simulink model "Simple_3_Model_C"  (R2022b)
settings: Solver=FixedStepAuto  StartTime=0.0  StopTime=1000  FixedStep=.05  RelTol=1e-3
libraries: realtime_pacer_lib x1, ros2lib x1
settings Model: Creator=hollis  LastModifiedBy=hunter
settings OptimizationCC: DefaultParameterBehavior=Inlined  EnhancedBackFolding=on  PassReuseOutputArgsAs=Individual arguments  ZeroExternalMemoryAtStartup=off  ZeroInternalMemoryAtStartup=off  OptimizeBlockOrder=speed  DifferentSizesBufferReuse=on  OptimizationCustomize=off  EfficientTunableParamExpr=on
settings DebuggingCC: ParameterTunabilityLossMsg=error
settings HardwareCC: TargetBitPerLong=64  TargetBitPerPointer=64  TargetBitPerSizeT=64  TargetBitPerPtrDiffT=64  TargetLongLongMode=on  TargetIntDivRoundTo=Zero  TargetEndianess=LittleEndian  TargetWordSize=64  TargetHWDeviceType=MATLAB Host  ProdEqTarget=off
settings ModelReferenceCC: EnableRefExpFcnMdlSchedulingChecks=on
settings SFSimCC: MATLABDynamicMemAlloc=off  SimTargetLang=C++
settings RTWCC: Description=Embedded Coder (host-based shared library target)  SystemTargetFile=ert_shrlib.tlc  TemplateMakefile=ert_default_tmf  Toolchain=GNU gcc/g++ | CMake/gmake (64-bit Linux)  BuildConfiguration=Release
settings CodeAppCC: ForceParamTrailComments=on  IgnoreCustomStorageClasses=off  OperatorAnnotations=on  SimulinkDataObjDesc=on  SFDataObjDesc=on  InsertBlockDesc=on
settings STFCustomTargetCC: TargetLangStandard=C99 (ISO)  MultiwordLength=256  GenerateSampleERTMain=on  ParMdlRefBuildCompliant=on  CompOptLevelCompliant=on  CombineOutputUpdateFcns=on  ERTCustomFileBanners=on  SupportNonInlinedSFcns=off  RemoveResetFunc=on  MATLABClassNameForMDSCustomization=Simulink.SoftwareTarget.ERTCustomization  ModelStepFunctionPrototypeControlCompliant=on  UseToolchainInfoCompliant=on  SystemTargetFile=ert_shrlib.tlc
settings ERTTargetCC: TargetLangStandard=C99 (ISO)  GenerateSampleERTMain=on  ConcurrentExecutionCompliant=off  SupportContinuousTime=on  CPPClassGenCompliant=off  InlinedParameterPlacement=NonHierarchical  ERTCustomFileTemplate=example_file_process.tlc

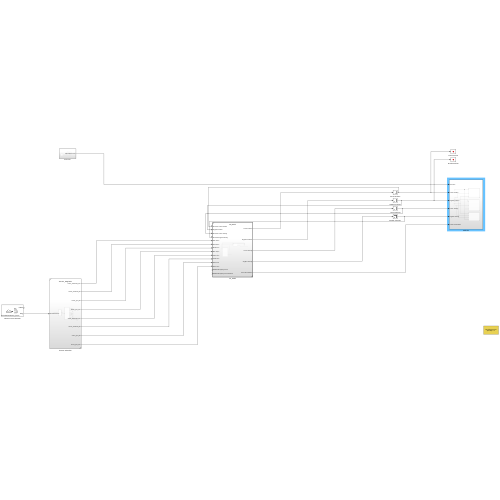
[thumbnail: Simulink's stored preview of the top-level diagram]
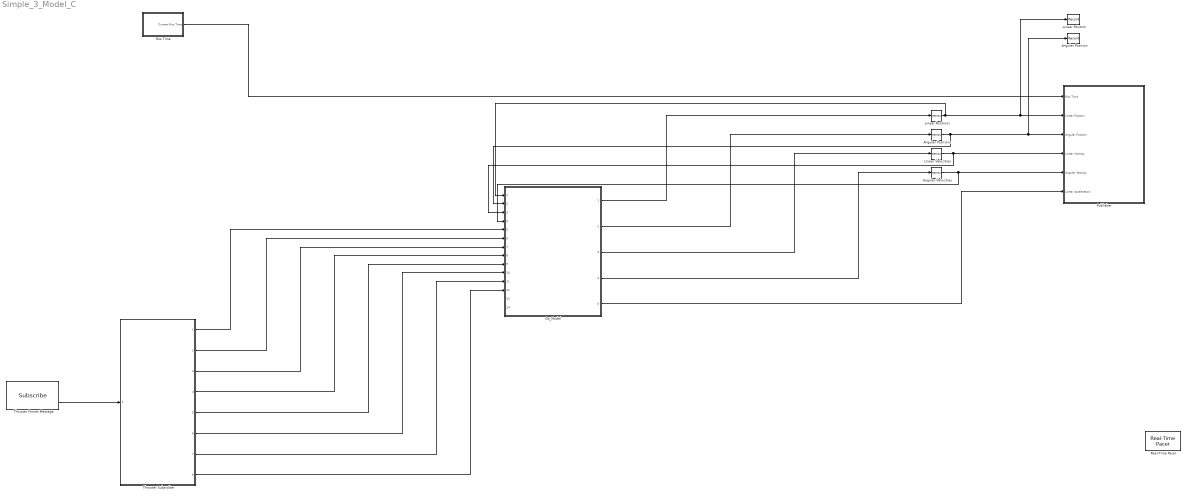
== system Simple_3_Model_C ==
  Angular Position : Record  FileSettingsInternal="{\"entries\":[{\"content\":{\"excelSettings\":{\"content\":{},\"type\":\"Streamout.ExcelSettings\"}},\"type\":\"Streamout.FileSettingStorage\",\"uuid\":\"5e6faace-5e05-446f-81ba-11f57939d993\"}],\"packageUris\":[\"http://schema.mathworks.com/mf0/streamout_blocks/R2020a\"],\"version\":\"1.0\"}"  SignalsInternal="{\"entries\":[{\"content\":{\"signals\":[{\"content\":{\"blockPath\":[\"Simple_3_Model_C/Angular Position\"],\"channel\":[],\"dimensions\":[1,3],\"domain\":\"Simple_3_Model_C/Angular Position\",\"hasChildren\":true,\"lineColor\":\"#b746ff\",\"plots\":[],\"port\":1,\"sid\":[],\"signalID\":309,\"signalName\":\"Angular Positions\"},\"type\":\"RecordBlkView.Signal\",\"uuid\":\"71cf2b88-9897-4e33-ab06-cf655d5c069d\"},{\"content\":{\"blockPath\":[\"Simple_3_Model_C/Angular Position\"],\"channel\":[1,1],\"dimensions\":[1,3],\"domain\":\"Simple_3_Model_C/Angular Position\",\"lineColor\":\"#d95319\",\"parentID\":309,\"plots\":[1],\"port\":1,\"sid\":[],\"signalID\":310,\"signalName\":\"Angular Positions\"},\"type\":\"RecordBlkView.Signal\",\"uuid\":\"81539e1a-8bab-4067-a60e-8d6090882496\"},{\"content\":{\"blockPath\":[\"Simple_3_Model_C/Angular Position\"],\"channel\":[1,2],\"dimensions\":[1,3],\"domain\":\"Simple_3_Model_C/Angular Position\",\"lineColor\":\"#d95319\",\"parentID\":309,\"plots\":[1],\"port\":1,\"sid\":[],\"signalID\":311,\"signalName\":\"Angular Positions\"},\"type\":\"RecordBlkView.Signal\",\"uuid\":\"9fdc422a-a8c8-4533-b613-6f9428fc65bd\"},{\"content\":{\"blockPath\":[\"Simple_3_Model_C/Angular Position\"],\"channel\":[1,3],\"dimensions\":[1,3],\"domain\":\"Simple_3_Model_C/Angular Position\",\"lineColor\":\"#edb120\",\"parentID\":309,\"plots\":[1],\"port\":1,\"sid\":[],\"signalID\":312,\"signalName\":\"Angular Positions\"},\"type\":\"RecordBlkView.Signal\",\"uuid\":\"9d0a805d-4d88-48d1-b17c-de63ad448efc\"}]},\"type\":\"RecordBlkView.InputSignals\",\"uuid\":\"3c6d1903-151d-4815-9e37-912ee027f4eb\"}],\"packageUris\":[\"http://schema.mathworks.com/mf0/streamout_blocks/R2020a\"],\"version\":\"1.0\"}"  VisualizationBindings="{\"sparklinesplugin\":{\"info\":[{\"bindingParametersList\":[],\"subplotID\":1}]}}"
  Angular Positions : Memory
  Angular Velocities : Memory
  Do_Model : Subsystem  TreatAsAtomicUnit=on  ReferencedSubsystem=Do_Model
  Linear Position : Record  FileSettingsInternal="{\"entries\":[{\"content\":{\"excelSettings\":{\"content\":{},\"type\":\"Streamout.ExcelSettings\"}},\"type\":\"Streamout.FileSettingStorage\",\"uuid\":\"9b40ccc1-229c-42d4-ab33-3394c1702d6d\"}],\"packageUris\":[\"http://schema.mathworks.com/mf0/streamout_blocks/R2020a\"],\"version\":\"1.0\"}"  SignalsInternal="{\"entries\":[{\"content\":{\"signals\":[{\"content\":{\"blockPath\":[\"Simple_3_Model_C/Linear Position\"],\"channel\":[],\"dimensions\":[1,3],\"domain\":\"Simple_3_Model_C/Linear Position\",\"hasChildren\":true,\"lineColor\":\"#ff13a6\",\"plots\":[],\"port\":1,\"sid\":[],\"signalID\":298,\"signalName\":\"Linear Positions\"},\"type\":\"RecordBlkView.Signal\",\"uuid\":\"238dd450-82a9-4540-9534-5454e0a4f67d\"},{\"content\":{\"blockPath\":[\"Simple_3_Model_C/Linear Position\"],\"channel\":[1,1],\"dimensions\":[1,3],\"domain\":\"Simple_3_Model_C/Linear Position\",\"lineColor\":\"#7e2f8e\",\"parentID\":298,\"plots\":[1],\"port\":1,\"sid\":[],\"signalID\":299,\"signalName\":\"Linear Positions\"},\"type\":\"RecordBlkView.Signal\",\"uuid\":\"0ffe9376-259a-4d51-9739-a81e551435e9\"},{\"content\":{\"blockPath\":[\"Simple_3_Model_C/Linear Position\"],\"channel\":[1,2],\"dimensions\":[1,3],\"domain\":\"Simple_3_Model_C/Linear Position\",\"lineColor\":\"#7e2f8e\",\"parentID\":298,\"plots\":[1],\"port\":1,\"sid\":[],\"signalID\":300,\"signalName\":\"Linear Positions\"},\"type\":\"RecordBlkView.Signal\",\"uuid\":\"2c7a0081-bf1d-46bd-8c42-e76470ee59e9\"},{\"content\":{\"blockPath\":[\"Simple_3_Model_C/Linear Position\"],\"channel\":[1,3],\"dimensions\":[1,3],\"domain\":\"Simple_3_Model_C/Linear Position\",\"lineColor\":\"#77ac30\",\"parentID\":298,\"plots\":[1],\"port\":1,\"sid\":[],\"signalID\":301,\"signalName\":\"Linear Positions\"},\"type\":\"RecordBlkView.Signal\",\"uuid\":\"79746674-a78a-4ff5-a75c-86a9df6f6110\"}]},\"type\":\"RecordBlkView.InputSignals\",\"uuid\":\"0a6c3fce-bcd9-43ed-9bd3-a9e2f38033f2\"}],\"packageUris\":[\"http://schema.mathworks.com/mf0/streamout_blocks/R2020a\"],\"version\":\"1.0\"}"  VisualizationBindings="{\"sparklinesplugin\":{\"info\":[{\"bindingParametersList\":[],\"subplotID\":1}]}}"
  Linear Positions : Memory  InitialCondition=[0.0,0.0,-1.0]
  Linear Velocities : Memory
  Publisher : Subsystem
  Real-Time Pacer : realtime_pacer_lib/Real-Time Pacer  simTimePerRealTime=1
  Ros Time : Subsystem
  Thruster Forces Message : ros2lib/Subscribe  topicSource=Specify your own  topic=/tempest/simulation/thruster_forces  messageType=std_msgs/Float32MultiArray  sampleTime=-1  QOSHistory=Keep last  QOSDepth=1  QOSReliability=Reliable  QOSDurability=Volatile
      settings: LibrarySourceBlock=roslib/ROS 2/Subscribe
  Thruster Subsrciber : Subsystem  ReferencedSubsystem=Thruster_Magnitude
  wires:
  Angular Velocities/1 -> Do_Model/4, Publisher/5(Angular Velocity)
  Linear Positions/1 -> Do_Model/1, Linear Position/1, Publisher/2(Linear Position)
  Linear Velocities/1 -> Do_Model/3, Publisher/4(Linear Velocity)
  Angular Positions/1 -> Do_Model/2, Angular Position/1, Publisher/3(Angular Position)
  Ros Time/1(Current Ros Time) -> Publisher/1(Ros Time)
  Thruster Forces Message/2 -> Thruster Subsrciber/1
  Thruster Subsrciber/1 -> Do_Model/5
  Thruster Subsrciber/2 -> Do_Model/6
  Thruster Subsrciber/3 -> Do_Model/7
  Thruster Subsrciber/4 -> Do_Model/8
  Thruster Subsrciber/5 -> Do_Model/9
  Thruster Subsrciber/6 -> Do_Model/10
  Thruster Subsrciber/7 -> Do_Model/11
  Thruster Subsrciber/8 -> Do_Model/12
  Do_Model/1 -> Linear Positions/1
  Do_Model/2 -> Angular Positions/1
  Do_Model/3 -> Linear Velocities/1
  Do_Model/4 -> Angular Velocities/1
  Do_Model/5 -> Publisher/6(Linear Acceleration)

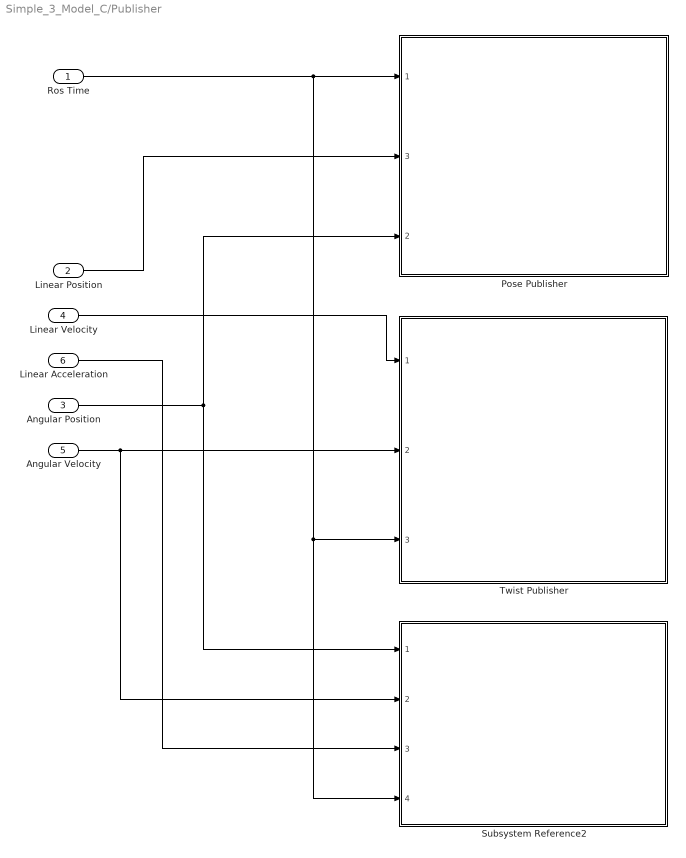
== system Simple_3_Model_C/Publisher ==
  Ros Time : Inport
  Linear Position : Inport  Port=2
  Angular Position : Inport  Port=3
  Linear Velocity : Inport  Port=4
  Angular Velocity : Inport  Port=5
  Linear Acceleration : Inport  Port=6
  Pose Publisher : Subsystem  ReferencedSubsystem=Pose_Publisher
      settings: PortSchema="{\"entries\":[{\"content\":{\"sides\":[{\"content\":{\"connectorIds\":[\"In1\",\"In3\",\"In2\"]},\"type\":\"ConnectorPlacement.EquallySpacedRectSide\",\"uuid\":\"18965d15-4955-4736-88eb-98a03933ea40\"},{\"content\":{\"connectorIds\":[],\"side\":\"RIGHT\"},\"type\":\"ConnectorPlacement.EquallySpacedRectSide\",\"uuid\":\"0239975c-7916-4f79-8798-13edb7247875\"},{\"content\":{\"connectorIds\":[],\"side\":\"TOP\"},\"type\":\"ConnectorPlacement.EquallySpacedRectSide\",\"uuid\":\"c7399201-5872-4101-b484-2a6e35d6576e\"}]},\"type\":\"ConnectorPlacement.EquallySpacedConnector\",\"uuid\":\"5ae7f81e-60af-4dbc-8d3d-d59049f94250\"}],\"packageUris\":[\"http://schema.mathworks.com/mf0/Connector/R2020b\"],\"version\":\"1.0\"}"
  Subsystem Reference2 : Subsystem  ReferencedSubsystem=Imu_Publisher
  Twist Publisher : Subsystem  ReferencedSubsystem=Twist_Publisher
  wires:
  Linear Position/1 -> Pose Publisher/3
  Linear Velocity/1 -> Twist Publisher/1
  Angular Position/1 -> Pose Publisher/2, Subsystem Reference2/1
  Angular Velocity/1 -> Subsystem Reference2/2, Twist Publisher/2
  Linear Acceleration/1 -> Subsystem Reference2/3
  Ros Time/1 -> Twist Publisher/3, Subsystem Reference2/4, Pose Publisher/1

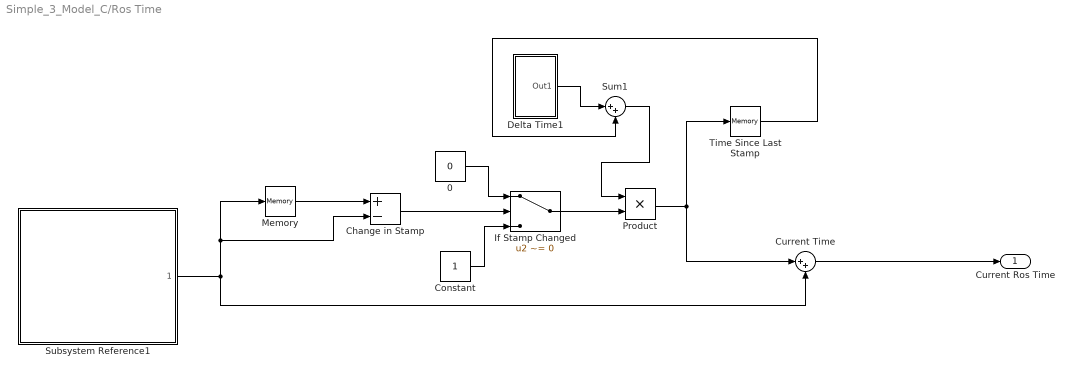
== system Simple_3_Model_C/Ros Time ==
  0 : Constant  Value=0
  Change in Stamp : Sum  Inputs=+-
  Constant : Constant
  Current Time : Sum  Inputs=|++
  Delta Time1 : Subsystem
  If Stamp Changed : Switch  Criteria=u2 ~= 0  SaturateOnIntegerOverflow=off  InputSameDT=off
  Memory : Memory
  Product : Product
  Subsystem Reference1 : Subsystem  ReferencedSubsystem=TimeSubscriber
  Sum1 : Sum  Inputs=|++
  Time Since Last Stamp : Memory
  Current Ros Time : Outport
  wires:
  Current Time/1 -> Current Ros Time/1
  Memory/1 -> Change in Stamp/1
  Constant/1 -> If Stamp Changed/3
  Delta Time1/1(Out1) -> Sum1/1
  Sum1/1 -> Product/1
  Time Since Last Stamp/1 -> Sum1/2
  Change in Stamp/1 -> If Stamp Changed/2
  If Stamp Changed/1 -> Product/2
  Product/1 -> Current Time/1, Time Since Last Stamp/1
  Subsystem Reference1/1 -> Change in Stamp/2, Memory/1, Current Time/2
  0/1 -> If Stamp Changed/1

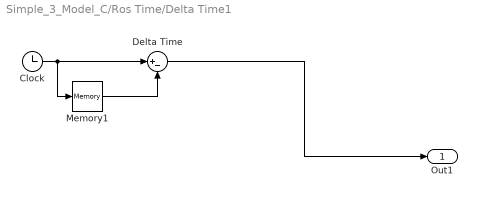
== system Simple_3_Model_C/Ros Time/Delta Time1 ==
  Clock : Clock
  Delta Time : Sum  Inputs=|+-
  Memory1 : Memory
  Out1 : Outport
  wires:
  Memory1/1 -> Delta Time/2
  Clock/1 -> Memory1/1, Delta Time/1
  Delta Time/1 -> Out1/1
